simulink model "HW6"  (R2018a)
settings: Solver=VariableStepAuto  StartTime=0.0  StopTime=500  RelTol=1e-3
settings Model: Creator=Sorawit Inprom  LastModifiedBy=Sorawit Inprom

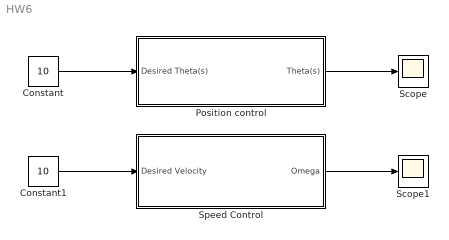
== system HW6 ==
  Constant : Constant  Value=10
  Constant1 : Constant  Value=10
  Position control : Subsystem  mask{kp=0.3/13, ki=0.2, kd=2, a=7, b=3}
      mask prompts: kp "Propotional Gain"; ki "Integral Gain"; kd "Derivative Gain"; a "constant a"; b "constant b"
  Scope : Scope
  Scope1 : Scope
  Speed Control : Subsystem  mask{kp=1, ki=1, a=7, b=3}
      mask prompts: kp "Propotional Gain"; ki "Integral Gain"; a "Constant a"; b "Constant b"
  wires:
  Constant/1 -> Position control/1(Desired Theta(s))
  Position control/1(Theta(s)) -> Scope/1
  Constant1/1 -> Speed Control/1(Desired Velocity)
  Speed Control/1(Omega) -> Scope1/1

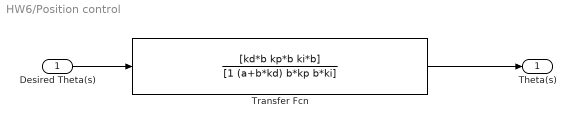
== system HW6/Position control ==
  Desired Theta(s) : Inport
  Transfer Fcn : TransferFcn  Numerator=[kd*b kp*b ki*b]  Denominator=[1 (a+b*kd) b*kp b*ki]
  Theta(s) : Outport
  wires:
  Transfer Fcn/1 -> Theta(s)/1
  Desired Theta(s)/1 -> Transfer Fcn/1

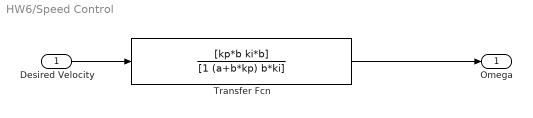
== system HW6/Speed Control ==
  Desired Velocity : Inport
  Transfer Fcn : TransferFcn  Numerator=[kp*b ki*b]  Denominator=[1 (a+b*kp) b*ki]
  Omega : Outport
  wires:
  Transfer Fcn/1 -> Omega/1
  Desired Velocity/1 -> Transfer Fcn/1
